simulink model "mbed_MAX11300"  (R2015a)
settings: Solver=FixedStepDiscrete  SolverMode=SingleTasking  StartTime=0.0  StopTime=50  FixedStep=1e-3  RelTol=1e-3
libraries: mbed_spi_max11300 x4, mbed_lib x1
settings Model: Creator=oh  LastModifiedBy=oh
settings OptimizationCC: OptimizeModelRefInitCode=on  LifeSpan=1
settings HardwareCC: ProdLargestAtomicInteger=Long  ProdLargestAtomicFloat=Double  ProdEndianess=LittleEndian  ProdHWDeviceType=ARM Compatible->ARM Cortex
settings RTWCC: SystemTargetFile=mbed.tlc  TemplateMakefile=mbed.tmf  Description=Mbed Target (Embedded Target)  TargetLang=C++
settings CodeAppCC: IgnoreCustomStorageClasses=off
settings STFCustomTargetCC: CombineOutputUpdateFcns=on  SupportContinuousTime=off  SupportVariableSizeSignals=off  SystemTargetFile=mbed.tlc
settings ERTTargetCC: SupportContinuousTime=off  SupportVariableSizeSignals=off  ERTCustomFileTemplate=mbed_file_process.tlc

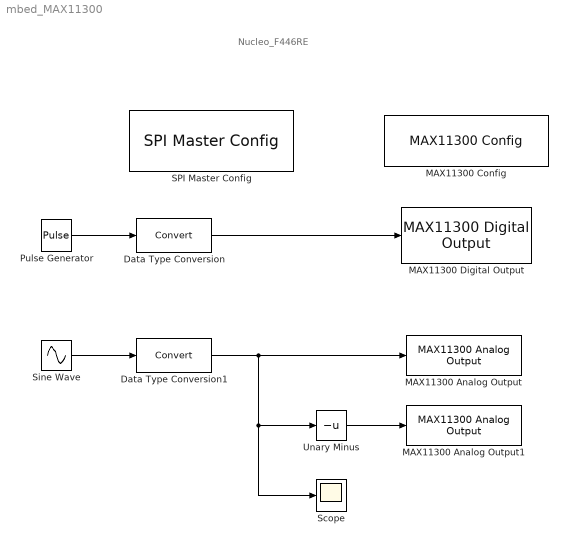
== system mbed_MAX11300 ==
  note: Nucleo_F446RE
  Data Type Conversion : DataTypeConversion
  Data Type Conversion1 : DataTypeConversion
  MAX11300 Analog Output : mbed_spi_max11300/MAX11300 Analog Output  CsPort=B  CsPin=6  Pin=1  Mode=relative  Range=0 to +10 V
  MAX11300 Analog Output1 : mbed_spi_max11300/MAX11300 Analog Output  CsPort=B  CsPin=6  Pin=2  Mode=relative  Range=0 to +10 V
  MAX11300 Config : mbed_spi_max11300/MAX11300 Config  Priority=1  SpiPort=1  CsPort=B  CsPin=6  AdcRate=200 kSPS  DacRef=Internal (2.5 V)  TempCh0=off  TempCh1=off  TempCh2=off
  MAX11300 Digital Output : mbed_spi_max11300/MAX11300 Digital Output  CsPort=B  CsPin=6  Pin=0  Level=4095
  Pulse Generator : DiscretePulseGenerator  PulseType=Time based  Period=4  PulseWidth=50
  SPI Master Config : mbed_lib/SPI/SPI Master Config  Priority=0  SpiPort=1  SpiFreq=100000  MosiPort=A  MosiPin=7  MisoPort=A  MisoPin=6  SclkPort=A  SclkPin=5
  Scope : Scope
  Sine Wave : Sin  Amplitude=0.5  Bias=0.5
  Unary Minus : UnaryMinus
  wires:
  Pulse Generator/1 -> Data Type Conversion/1
  Data Type Conversion/1 -> MAX11300 Digital Output/1
  Sine Wave/1 -> Data Type Conversion1/1
  Unary Minus/1 -> MAX11300 Analog Output1/1
  Data Type Conversion1/1 -> MAX11300 Analog Output/1, Unary Minus/1, Scope/1
